simulink model "C01A_DC_MotorEquation"  (R2024b)
settings: Solver=VariableStepAuto  StartTime=0.0  StopTime=0.2  RelTol=1e-3
undefined symbols (not defined in the file): b, J, Km, L, R, RadToRpm
settings Model: Creator=Davide  LastModifiedBy=Utente
settings DataIOCC: ReturnWorkspaceOutputs=off
settings OptimizationCC: ReuseModelBlockBuffer=off
settings RTWCC: GPUComputeCapability=3.5

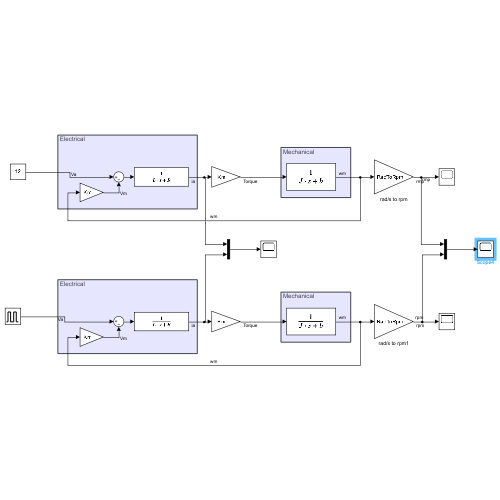
[thumbnail: Simulink's stored preview of the top-level diagram]
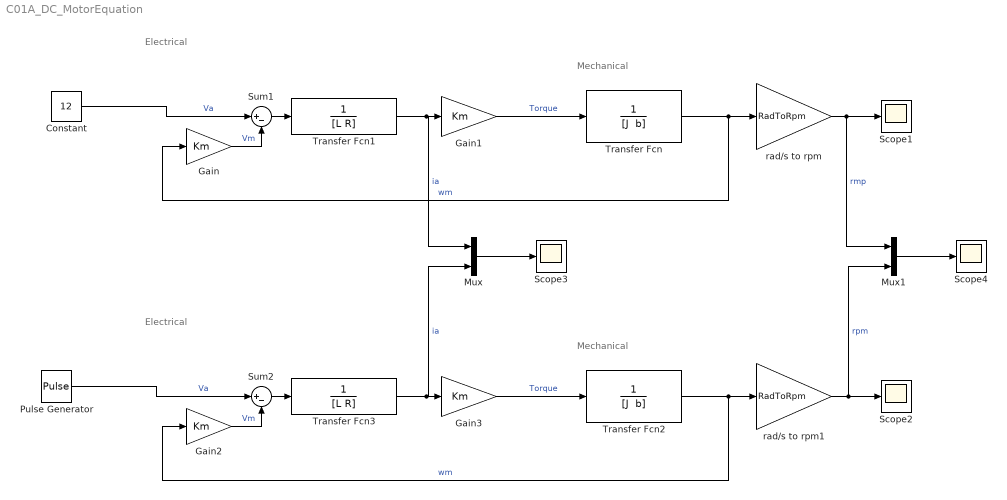
== system C01A_DC_MotorEquation ==
  note: Electrical
  note: Mechanical
  note: Mechanical
  note: Electrical
  Constant : Constant  Value=12
  Gain{,1..3} (4 alike) : Gain  Gain=Km
  Mux : Mux  Inputs=2
  Mux1 : Mux  Inputs=2
  Pulse Generator : DiscretePulseGenerator  PulseType=Time based  Amplitude=24  Period=0.001  PulseWidth=50
  Scope{1..4} (4 alike) : Scope
  Sum1 : Sum  Inputs=|+-
  Sum2 : Sum  Inputs=|+-
  Transfer Fcn : TransferFcn  Denominator="[J  b]"
  Transfer Fcn1 : TransferFcn  Denominator=[L R]
  Transfer Fcn2 : TransferFcn  Denominator="[J  b]"
  Transfer Fcn3 : TransferFcn  Denominator=[L R]
  rad/s to rpm : Gain  Gain=RadToRpm  SaturateOnIntegerOverflow=on  OutDataTypeStr=Inherit: Same as input  ParamDataTypeStr=Inherit: Same as input
  rad/s to rpm1 : Gain  Gain=RadToRpm  SaturateOnIntegerOverflow=on  OutDataTypeStr=Inherit: Same as input  ParamDataTypeStr=Inherit: Same as input
  wires:
  Transfer Fcn/1 -> rad/s to rpm/1, Gain/1  "wm"
  Transfer Fcn1/1 -> Mux/1, Gain1/1  "ia"
  Sum1/1 -> Transfer Fcn1/1
  Gain/1 -> Sum1/2  "Vm"
  Constant/1 -> Sum1/1  "Va"
  Gain1/1 -> Transfer Fcn/1  "Torque"
  Gain3/1 -> Transfer Fcn2/1  "Torque"
  Transfer Fcn2/1 -> rad/s to rpm1/1, Gain2/1  "wm"
  Sum2/1 -> Transfer Fcn3/1
  Pulse Generator/1 -> Sum2/1  "Va"
  Transfer Fcn3/1 -> Mux/2, Gain3/1  "ia"
  Gain2/1 -> Sum2/2  "Vm"
  Mux/1 -> Scope3/1
  rad/s to rpm/1 -> Mux1/1, Scope1/1  "rmp"
  rad/s to rpm1/1 -> Mux1/2, Scope2/1  "rpm"
  Mux1/1 -> Scope4/1
